simulink model "Mod3_4"  (Simulink 7.4)
settings: Solver=FixedStepDiscrete  SolverMode=SingleTasking  StartTime=0.0  StopTime=1  FixedStep=1/Fs  MaxStep=1e-6  RelTol=1e-3  AbsTol=1e-6
InitFcn:
  | Enable_Errors =0;
  | 
  | Alpha_ = Enable_Errors*[1e-3 1e-3 1e-3];        % integrator gain errors
  | Beta_  =  Enable_Errors*[ 1e-4  1e-4   1e-4];      % integrator pole error
  | 
  | if Enable_Errors==1
  |      C_gain = 1e5;   % comparitor gain
  | else
  |      C_gain=1e12;
  | end;
  | 
  | Fs_out = 100e3;   % output sample rate
  | OSR=64;               % input oversampling factor
  | Fs=OSR*Fs_out;   %  input sampling rate
undefined symbols (not defined in the file or in its folder): One, sided
libraries: simulink x4, dspbuff3 x3, dspsnks4 x2, dspmlti4 x2, dspspect3 x2, commsynccomp2 x1, dsparch4 x1, dspadpt3 x1, dspobslib x1, dspsigops x1, dspstat3 x1
settings Model: Creator=don  LastModifiedBy=Dick  ExtModeTrigMode=oneshot  ExtModeArmWhenConnect=off
settings DataIOCC: LimitDataPoints=off  SaveOutput=off  SaveTime=off  SignalLoggingName=sigsOut
settings OptimizationCC: BlockReduction=off  BooleanDataType=off  InitFltsAndDblsToZero=on
settings DebuggingCC: SaveWithParameterizedLinksMsg=none  SignalResolutionControl=TryResolveAllWithWarning  SolverPrmCheckMsg=none  MultiTaskDSMMsg=warning  MultiTaskCondExecSysMsg=none  IntegerOverflowMsg=none  StrictBusMsg=None
settings HardwareCC: TargetUnknown=on
settings RTWCC: IncludeERTFirstTime=on
settings GRTTargetCC: TargetFcnLib=ansi_tfl_tmw.mat

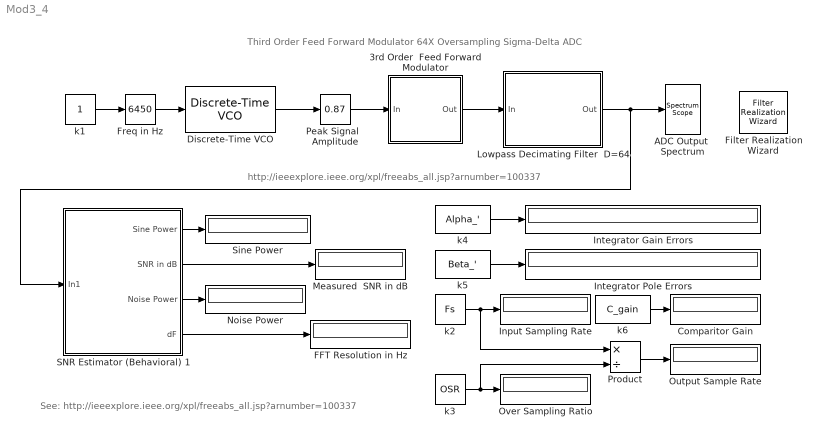
== system Mod3_4 ==
  note: Third Order Feed Forward Modulator
      | 64X Oversampling Sigma-Delta ADC
  note: http://ieeexplore.ieee.org/xpl/freeabs_all.jsp?arnumber=100337
  note: See: http://ieeexplore.ieee.org/xpl/freeabs_all.jsp?arnumber=100337
  3rd Order  Feed Forward Modulator : Subsystem
  ADC Output  Spectrum : dspsnks4/Spectrum Scope  DialogController=dspdialog.SpectrumScope  DialogControllerArgs=DataTag0  SystemSampleTime=-1  ScopeProperties=off  Domain=Frequency  HorizSpan=1  UseBuffer=on  BufferSize=1024  Overlap=0  inpFftLenInherit=off  FFTlength=128  numAvg=1  DisplayProperties=off  AxisGrid=on  Memory=off  FrameNumber=on  AxisLegend=off  AxisZoom=off  OpenScopeAtSimStart=on  OpenScopeImmediately=off  FigPos=[80 61 319 232]  AxisProperties=on  XUnits=Hertz  XRange=One-sided ([0...Fs/2])  XDisplay=0  InheritXIncr=on  XIncr=1.0  XLabel=Samples  XLimit=User-defined  YUnits=dBW  XMax=Fs/(2*OSR)  XMin=0  YLabel=Magnitude, dB  LineProperties=off  wintypeSpecScope=Hann  RsSpecScope=50  betaSpecScope=5  winsampSpecScope=Periodic  XAxisParamsVer=6.9
      settings: YMin=-200  YMax=0
  Comparitor Gain : Display
      settings: Decimation=1000
  Discrete-Time VCO : commsynccomp2/Discrete-Time VCO  SystemSampleTime=-1  Ac=1  Fc=0  Kc=1  Ph=0  ts=1/Fs
  FFT Resolution in Hz : Display
  Filter Realization Wizard : dsparch4/Filter Realization Wizard  SystemSampleTime=-1
  Freq in Hz : simulink/Math Operations/Slider Gain  SystemSampleTime=-1  low=0  gain=6450  high=20000
  Input Sampling Rate : Display
      settings: Decimation=1000
  Integrator Gain Errors : Display
      settings: Decimation=1000
  Integrator Pole Errors : Display
      settings: Decimation=1000
  Lowpass Decimating Filter  D=64 : Subsystem  Tag=BlockMethodSubSystem
  Measured  SNR in dB : Display
  Noise Power : Display
  Output Sample Rate : Display
      settings: Decimation=1000
  Over Sampling Ratio : Display
      settings: Decimation=1000
  Peak Signal   Amplitude : simulink/Math Operations/Slider Gain  SystemSampleTime=-1  low=0  gain=0.87  high=1
  Product : Product  Inputs=*/  OutDataType=fixdt(1, 16)  OutScaling=2^0  RndMeth=Zero
  SNR Estimator (Behavioral) 1 : Subsystem  mask{Frame=256, Pcnt_Nyquist=100, Navg=1, Ymax=-50, Ymin=-140, Hold_Off=260, ON_FFT_LINE=off}
      mask prompts: Frame "Input Frame Size"; Pcnt_Nyquist "Percentage of Fs/2 to use in noise power measurement"; Navg "Number of Averages"; Ymax "Noise Plot Ymax in dB"; Ymin "Noise Plot Ymin in dB"; Hold_Off "Calculation Hold Off in SAMPLES"; ON_FFT_LINE "Check this box if the signal is on an FFT Analysis Line."
      mask Display:
      | disp('SNR \n Measurement')
      | port_label('Input',1,'In')
      | port_label('Output',1,'Sine Power')
      | port_label('Output',2,'SNR in dB')
      | port_label('Output',3,'Noise Power')
      | port_label('Output',4,'FFT Line Freq')
  "Sine Power " : Display
  k1 : Constant  OutDataType=fixdt(1, 16)  OutScaling=2^0
  k2 : Constant  Value=Fs  OutDataType=fixdt(1, 16)  OutScaling=2^0
  k3 : Constant  Value=OSR  OutDataType=fixdt(1, 16)  OutScaling=2^0
  k4 : Constant  Value=Alpha_'  OutDataType=fixdt(1, 16)  OutScaling=2^0
  k5 : Constant  Value=Beta_'  OutDataType=fixdt(1, 16)  OutScaling=2^0
  k6 : Constant  Value=C_gain  OutDataType=fixdt(1, 16)  OutScaling=2^0
  wires:
  Discrete-Time VCO/1 -> Peak Signal   Amplitude/1
  Peak Signal   Amplitude/1 -> 3rd Order  Feed Forward Modulator/1(In)
  Freq in Hz/1 -> Discrete-Time VCO/1
  k1/1 -> Freq in Hz/1
  k3/1 -> Over Sampling Ratio/1, Product/2
  Product/1 -> Output Sample Rate/1
  Lowpass Decimating Filter  D=64/1(Out) -> ADC Output  Spectrum/1, SNR Estimator (Behavioral) 1/1(In1)
  SNR Estimator (Behavioral) 1/2(SNR in dB) -> Measured  SNR in dB/1
  SNR Estimator (Behavioral) 1/1(Sine Power) -> "Sine Power "/1
  SNR Estimator (Behavioral) 1/3(Noise Power) -> Noise Power/1
  SNR Estimator (Behavioral) 1/4(dF) -> FFT Resolution in Hz/1
  3rd Order  Feed Forward Modulator/1(Out) -> Lowpass Decimating Filter  D=64/1(In)
  k4/1 -> Integrator Gain Errors/1
  k5/1 -> Integrator Pole Errors/1
  k6/1 -> Comparitor Gain/1
  k2/1 -> Input Sampling Rate/1, Product/1

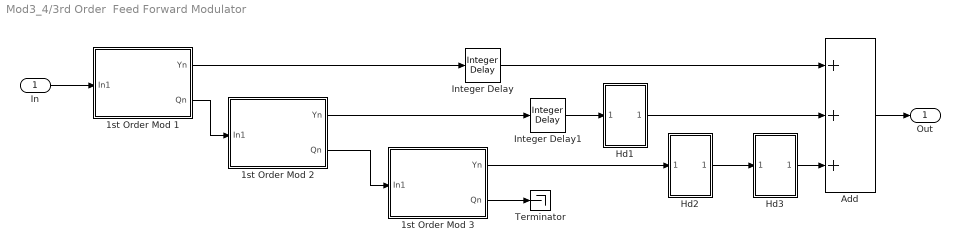
== system Mod3_4/3rd Order  Feed Forward Modulator ==
  In : Inport
  1st Order Mod 1 : Subsystem
  1st Order Mod 2 : Subsystem
  1st Order Mod 3 : Subsystem
  Add : Sum  Inputs=+++  OutDataType=fixdt(1, 16)  OutScaling=2^-10
  Hd1 : Subsystem
  Hd2 : Subsystem
  Hd3 : Subsystem
  Integer Delay : simulink/Discrete/Integer Delay  vinit=0.0  samptime=-1  NumDelays=2
  Integer Delay1 : simulink/Discrete/Integer Delay  vinit=0.0  samptime=-1  NumDelays=1
  Terminator : Terminator
  Out : Outport
  wires:
  1st Order Mod 1/2(Qn) -> 1st Order Mod 2/1(In1)
  1st Order Mod 2/2(Qn) -> 1st Order Mod 3/1(In1)
  1st Order Mod 1/1(Yn) -> Integer Delay/1
  Add/1 -> Out/1
  In/1 -> 1st Order Mod 1/1(In1)
  1st Order Mod 3/2(Qn) -> Terminator/1
  1st Order Mod 2/1(Yn) -> Integer Delay1/1
  Hd1/1(Out1) -> Add/2
  1st Order Mod 3/1(Yn) -> Hd2/1(In1)
  Hd2/1(Out1) -> Hd3/1(In1)
  Hd3/1(Out1) -> Add/3
  Integer Delay1/1 -> Hd1/1(In1)
  Integer Delay/1 -> Add/1

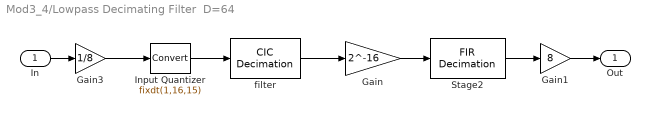
== system Mod3_4/Lowpass Decimating Filter  D=64 ==
  In : Inport
  Gain : Gain  Gain=2^-16  ParameterDataType=fixdt(1, 16)  ParameterScaling=2^0  OutDataTypeMode=double  OutDataType=fixdt(1, 16)  OutScaling=2^0  OutDataTypeStr=double
  Gain1 : Gain  Gain=8  ParameterDataType=fixdt(1, 16)  ParameterScaling=2^0  OutDataType=fixdt(1, 16)  OutScaling=2^0
  Gain3 : Gain  Gain=1/8  ParameterDataType=fixdt(1, 16)  ParameterScaling=2^0  OutDataType=fixdt(1, 16)  OutScaling=2^0
  Input Quantizer : DataTypeConversion  OutDataTypeMode=Specify via dialog  OutDataType=fixdt(1,16,15)  OutDataTypeStr=fixdt(1,16,15)  RndMeth=Round  SaturateOnIntegerOverflow=on
  Stage2 : dspmlti4/FIR Decimation  Tag=BlockMethodSubSystem  DialogController=dspdialog.FIRDecimation  DialogControllerArgs=DataTag1  h=[-1.03672832769806e-005 -2.30043872918871e-005 -3.81607660571471e-005 -4.73451966989753e-005 -4.15314840476983e-005 -1.53294381464531e-005 2.81247599902108e-005 7.548106001899e-005 0.000106956615554732 0.000105170685159055 6.53313671878897e-005 1.10615621617923e-006 -5.84899984530656e-005 -8.16995174647979e-005 -5.10738247202842e-005 2.39521887480776e-005 0.000107288371406307 0.000151796841211863 0.000124298000926512 2.72100582090589e-005 -9.64877715240933e-005 -0.000180990434728796 -0.00017184528528019 -5.94684973243738e-005 0.000107769129196385 0.000242056255586363 0.000260704715966674 0.00013493651668018 -8.5000049815582e-005 -0.000286841516056665 -0.000352051709584436 -0.000223619051276749 5.19058171754285e-005 0.000336492393063494 0.000467639101393255 0.000349059309073545 1.54942235654423e-005 -0.000369695852959625 -0.000591913524331285 -0.000502692833274323 -0.000114059879575764 0.000387970305599598 0.00072897644788482 0.000693620406886893 0.000257154373538894 -0.000377310868830626 -0.00086882045273623 -0.000918947560229279 -0.000448725221904726 0.000330696351510504 0.00100679796943566 0.00118065668729705 0.000698048038921545 -0.00023505915729049 -0.00113201638035961 -0.00147528588722154 -0.00101064908239849 7.91467137436565e-005 0.00123408252213311 0.00179975815120012 0.00139348389465366 0.000151247519594855 -0.00129860929748089 -0.00214716507990412 -0.00185109070890518 -0.000469898879291989 0.00131013209846719 0.00250931405838737 0.00238792045365338 0.000892372059188557 -0.00125000870520108 -0.00287487459601245 -0.00300688117971149 -0.00143501818412447 0.00109708430001496 0.00322994871994394 0.00371003867432686 0.00211584322619809 -0.000826876587517894 -0.00355768687459038 -0.00449894643382303 -0.00295548408089549 0.000410455632566669 0.00383775807505308 0.0053752440064593 0.00397885063139594 0.000187407314825939 -0.00404552680663259 -0.00634177196701517 -0.00521802991372615 -0.00101148845885873 0.00415062606771981 0.00740459885236922 0.00671755764137374 0.00212208484585908 -0.00411422714989155 -0.00857666811063853 -0.00854431755242137 -0.00360667248328686 0.00388301665917001 0.0098836881541225 0.0108056935767939 0.0056020971184406 -0.00337754872457966 -0.0113763732976555 -0.0136877273059045 -0.00834263488466605 0.00246546701482214 0.0131561884005966 0.0175416995656231 0.012273978356376 -0.000894329941755317 -0.0154384118477508 -0.0231117442236786 -0.0183702494962771 -0.00191023855567135 0.0187347462761574 0.0322678072014156 0.0292453606752335 0.00763813070524675 -0.0245476659764372 -0.0513189673918339 -0.0550085939173135 -0.0243158330095173 0.0395342433994632 0.121541322450517 0.197564379590681 0.24318839888947 0.24318839888947 0.197564379590681 0.121541322450517 0.0395342433994632 -0.0243158330095173 -0.0550085939173135 -0.0513189673918339 -0.0245476659764372 0.00763813070524675 0.0292453606752335 0.0322678072014156 0.0187347462761574 -0.00191023855567135 -0.0183702494962771 -0.0231117442236786 -0.0154384118477508 -0.000894329941755317 0.012273978356376 0.0175416995656231 0.0131561884005966 0.00246546701482214 -0.00834263488466605 -0.0136877273059045 -0.0113763732976555 -0.00337754872457966 0.0056020971184406 0.0108056935767939 0.0098836881541225 0.00388301665917001 -0.00360667248328686 -0.00854431755242137 -0.00857666811063853 -0.00411422714989155 0.00212208484585908 0.00671755764137374 0.00740459885236922 0.00415062606771981 -0.00101148845885873 -0.00521802991372615 -0.00634177196701517 -0.00404552680663259 0.000187407314825939 0.00397885063139594 0.0053752440064593 0.00383775807505308 0.000410455632566669 -0.00295548408089549 -0.00449894643382303 -0.00355768687459038 -0.000826876587517894 0.00211584322619809 0.00371003867432686 0.00322994871994394 0.00109708430001496 -0.00143501818412447 -0.00300688117971149 -0.00287487459601245 -0.00125000870520108 0.000892372059188557 0.00238792045365338 0.00250931405838737 0.00131013209846719 -0.000469898879291989 -0.00185109070890518 -0.00214716507990412 -0.00129860929748089 ...(+1336 chars)]  D=4  filtStruct=Direct form  framing=Maintain input frame size  outputBufInitCond=0  roundingMode=Floor  overflowMode=off  FilterSource=Specify via dialog  FilterObject=Hm_firdecim
  filter : dspmlti4/CIC Decimation  DialogController=dspdialog.CICDecimation  filtFrom=Dialog  filtobj=Hm_decim  ftype=Decimator  R=16  M=1  N=4  filterInternals=Full precision  BPS=[32 32 32 32 32 32 32 32]  FLPS=[15 15 15 15 15 15 15 15]  outputWordLength=32  outputFracLength=15  launchFVT=off  framing=Maintain input frame rate
  Out : Outport
  wires:
  In/1 -> Gain3/1
  filter/1 -> Gain/1
  Stage2/1 -> Gain1/1
  Gain/1 -> Stage2/1
  Gain1/1 -> Out/1
  Gain3/1 -> Input Quantizer/1
  Input Quantizer/1 -> filter/1

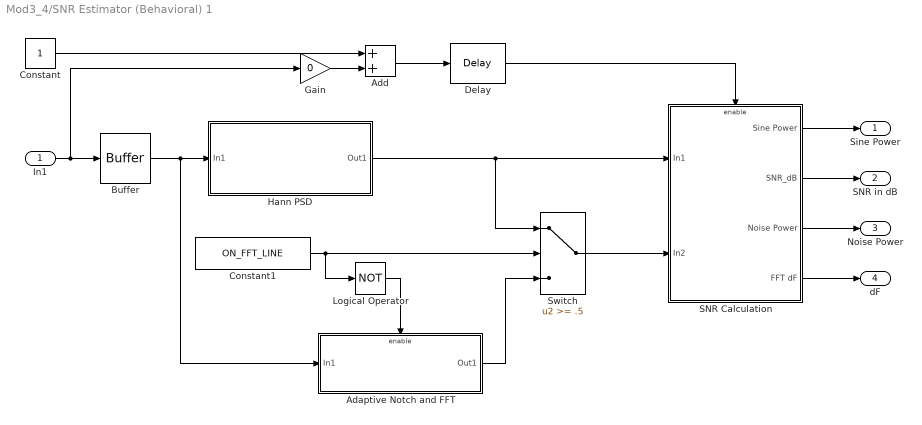
== system Mod3_4/SNR Estimator (Behavioral) 1 ==
  In1 : Inport
  Adaptive Notch and FFT : Subsystem  TreatAsAtomicUnit=on
  Add : Sum  OutDataType=fixdt(1, 16)  OutScaling=2^-10
  Buffer : dspbuff3/Buffer  N=Frame  V=0  ic=0
  Constant : Constant  OutDataType=fixdt(1, 16)  OutScaling=2^0
  Constant1 : Constant  Value=ON_FFT_LINE  OutDataTypeMode=boolean  OutDataType=fixdt(1, 16)  OutScaling=2^0  OutDataTypeStr=boolean
  Delay : dspsigops/Delay  dly_unit=Samples  delay=Hold_Off  ic_detail=off  dif_ic_for_ch=off  dif_ic_for_dly=off  ic=0  reset_popup=None
  Gain : Gain  Gain=0  ParameterDataType=fixdt(1, 16)  ParameterScaling=2^0  OutDataType=fixdt(1, 16)  OutScaling=2^0
  Hann PSD : Subsystem
  Logical Operator : Logic  Operator=NOT  AllPortsSameDT=off  OutDataTypeMode=boolean  LogicDataType=fixdt(0, 8)  OutDataTypeStr=boolean
  SNR Calculation : Subsystem
  Switch : Switch  Threshold=.5  OutDataType=fixdt(1, 16)  OutScaling=2^0
  Sine Power : Outport
  SNR in dB : Outport  Port=2
  Noise Power : Outport  Port=3
  dF : Outport  Port=4
  wires:
  In1/1 -> Buffer/1, Gain/1
  SNR Calculation/2(SNR_dB) -> SNR in dB/1
  Hann PSD/1(Out1) -> SNR Calculation/1(In1), Switch/1
  Buffer/1 -> Hann PSD/1(In1), Adaptive Notch and FFT/1(In1)
  SNR Calculation/1(Sine Power) -> Sine Power/1
  Switch/1 -> SNR Calculation/2(In2)
  SNR Calculation/3(Noise Power) -> Noise Power/1
  Delay/1 -> SNR Calculation/Enable
  Adaptive Notch and FFT/1(Out1) -> Switch/3
  Constant1/1 -> Switch/2, Logical Operator/1
  Logical Operator/1 -> Adaptive Notch and FFT/Enable
  SNR Calculation/4(FFT dF) -> dF/1
  Add/1 -> Delay/1
  Constant/1 -> Add/1
  Gain/1 -> Add/2

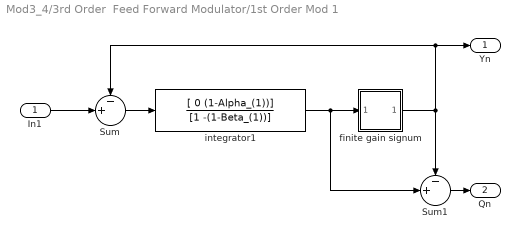
== system Mod3_4/3rd Order  Feed Forward Modulator/1st Order Mod 1 ==
  In1 : Inport
  Sum : Sum  Inputs=-+|  OutDataType=sfix(16)  OutScaling=2^0  SaturateOnIntegerOverflow=on  InputSameDT=on  OutDataTypeStr=Inherit: Same as first input
  Sum1 : Sum  Inputs=-+|  OutDataType=sfix(16)  OutScaling=2^0  SaturateOnIntegerOverflow=on  InputSameDT=on  OutDataTypeStr=Inherit: Same as first input
  "finite gain signum " : Subsystem  AncestorBlock=rab_favorites/non linear (real)  mask{alpha=C_gain}
      mask init:
      | x=-3:0.05:3;  y= tanh(alpha*x);
      mask Display: plot(x,y)
  integrator1 : DiscreteFilter  Numerator=[ 0 (1-Alpha_(1))]  Denominator=[1 -(1-Beta_(1))]
  Yn : Outport
  Qn : Outport  Port=2
  wires:
  Sum/1 -> integrator1/1
  integrator1/1 -> Sum1/2, "finite gain signum "/1(In1)
  Sum1/1 -> Qn/1
  "finite gain signum "/1(Out1) -> Sum1/1, Sum/1, Yn/1
  In1/1 -> Sum/2

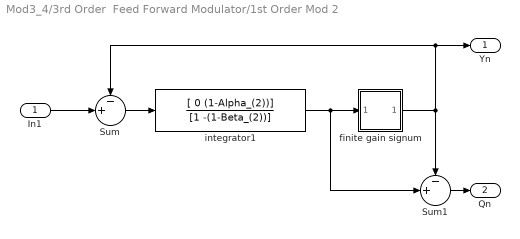
== system Mod3_4/3rd Order  Feed Forward Modulator/1st Order Mod 2 ==
  In1 : Inport
  Sum : Sum  Inputs=-+|  OutDataType=sfix(16)  OutScaling=2^0  SaturateOnIntegerOverflow=on  InputSameDT=on  OutDataTypeStr=Inherit: Same as first input
  Sum1 : Sum  Inputs=-+|  OutDataType=sfix(16)  OutScaling=2^0  SaturateOnIntegerOverflow=on  InputSameDT=on  OutDataTypeStr=Inherit: Same as first input
  "finite gain signum " : Subsystem  AncestorBlock=rab_favorites/non linear (real)  mask{alpha=C_gain}
      mask init:
      | x=-3:0.05:3;  y= tanh(alpha*x);
      mask Display: plot(x,y)
  integrator1 : DiscreteFilter  Numerator=[ 0 (1-Alpha_(2))]  Denominator=[1 -(1-Beta_(2))]
  Yn : Outport
  Qn : Outport  Port=2
  wires:
  In1/1 -> Sum/2
  "finite gain signum "/1(Out1) -> Yn/1, Sum/1, Sum1/1
  Sum1/1 -> Qn/1
  integrator1/1 -> "finite gain signum "/1(In1), Sum1/2
  Sum/1 -> integrator1/1

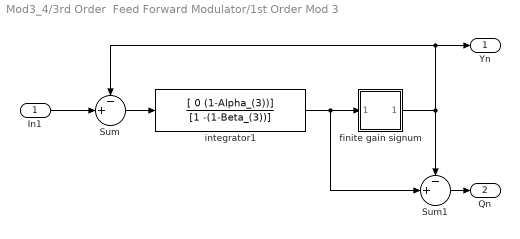
== system Mod3_4/3rd Order  Feed Forward Modulator/1st Order Mod 3 ==
  In1 : Inport
  Sum : Sum  Inputs=-+|  OutDataType=sfix(16)  OutScaling=2^0  SaturateOnIntegerOverflow=on  InputSameDT=on  OutDataTypeStr=Inherit: Same as first input
  Sum1 : Sum  Inputs=-+|  OutDataType=sfix(16)  OutScaling=2^0  SaturateOnIntegerOverflow=on  InputSameDT=on  OutDataTypeStr=Inherit: Same as first input
  "finite gain signum " : Subsystem  AncestorBlock=rab_favorites/non linear (real)  mask{alpha=C_gain}
      mask init:
      | x=-3:0.05:3;  y= tanh(alpha*x);
      mask Display: plot(x,y)
  integrator1 : DiscreteFilter  Numerator=[ 0 (1-Alpha_(3))]  Denominator=[1 -(1-Beta_(3))]
  Yn : Outport
  Qn : Outport  Port=2
  wires:
  Sum/1 -> integrator1/1
  integrator1/1 -> Sum1/2, "finite gain signum "/1(In1)
  Sum1/1 -> Qn/1
  "finite gain signum "/1(Out1) -> Sum1/1, Sum/1, Yn/1
  In1/1 -> Sum/2

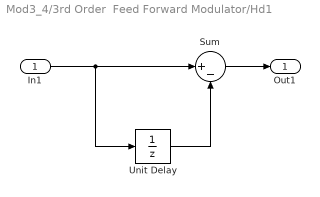
== system Mod3_4/3rd Order  Feed Forward Modulator/Hd1 ==
  In1 : Inport
  Sum : Sum  Inputs=|+-  OutDataType=sfix(16)  OutScaling=2^0  SaturateOnIntegerOverflow=on  InputSameDT=on  OutDataTypeStr=Inherit: Same as first input
  Unit Delay : UnitDelay  SampleTime=-1
  Out1 : Outport
  wires:
  In1/1 -> Sum/1, Unit Delay/1
  Sum/1 -> Out1/1
  Unit Delay/1 -> Sum/2

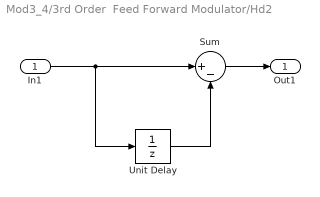
== system Mod3_4/3rd Order  Feed Forward Modulator/Hd2 ==
  In1 : Inport
  Sum : Sum  Inputs=|+-  OutDataType=sfix(16)  OutScaling=2^0  SaturateOnIntegerOverflow=on  InputSameDT=on  OutDataTypeStr=Inherit: Same as first input
  Unit Delay : UnitDelay  SampleTime=-1
  Out1 : Outport
  wires:
  Unit Delay/1 -> Sum/2
  Sum/1 -> Out1/1
  In1/1 -> Unit Delay/1, Sum/1

== system Mod3_4/3rd Order  Feed Forward Modulator/Hd3 ==
  In1 : Inport
  Sum : Sum  Inputs=|+-  OutDataType=sfix(16)  OutScaling=2^0  SaturateOnIntegerOverflow=on  InputSameDT=on  OutDataTypeStr=Inherit: Same as first input
  Unit Delay : UnitDelay  SampleTime=-1
  Out1 : Outport
  wires:
  In1/1 -> Sum/1, Unit Delay/1
  Sum/1 -> Out1/1
  Unit Delay/1 -> Sum/2

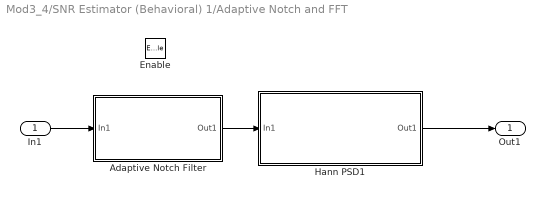
== system Mod3_4/SNR Estimator (Behavioral) 1/Adaptive Notch and FFT ==
  In1 : Inport  OutDataType=fixdt(1, 16)  OutScaling=2^0
  Enable : EnablePort
  Adaptive Notch Filter : Subsystem
  Hann PSD1 : Subsystem
  Out1 : Outport  OutDataType=fixdt(1, 16)  OutScaling=2^0
  wires:
  Adaptive Notch Filter/1(Out1) -> Hann PSD1/1(In1)
  Hann PSD1/1(Out1) -> Out1/1
  In1/1 -> Adaptive Notch Filter/1(In1)

== system Mod3_4/SNR Estimator (Behavioral) 1/Hann PSD ==
  note: Real Data produces a perfectly
      | symmetrical spectrum.
      | Use 1/2 of it.
  In1 : Inport
  Periodogram using  Hann Window : dspspect3/Periodogram  SystemSampleTime=-1  measurement=Mean-square spectrum  wintype=Hann  Rs=RsSpecScope  beta=betaSpecScope  winsamp=Periodic  inheritFFT=on  fftsize=FFTlength  navg=Navg  inheritTs=on  Ts=1
  Selector : Selector  InputPortWidth=Frame  IndexOptions=Index vector (dialog)  Indices=[1: Frame/2]  OutputSizes=1
  Out1 : Outport
  wires:
  Selector/1 -> Out1/1
  Periodogram using  Hann Window/1 -> Selector/1
  In1/1 -> Periodogram using  Hann Window/1

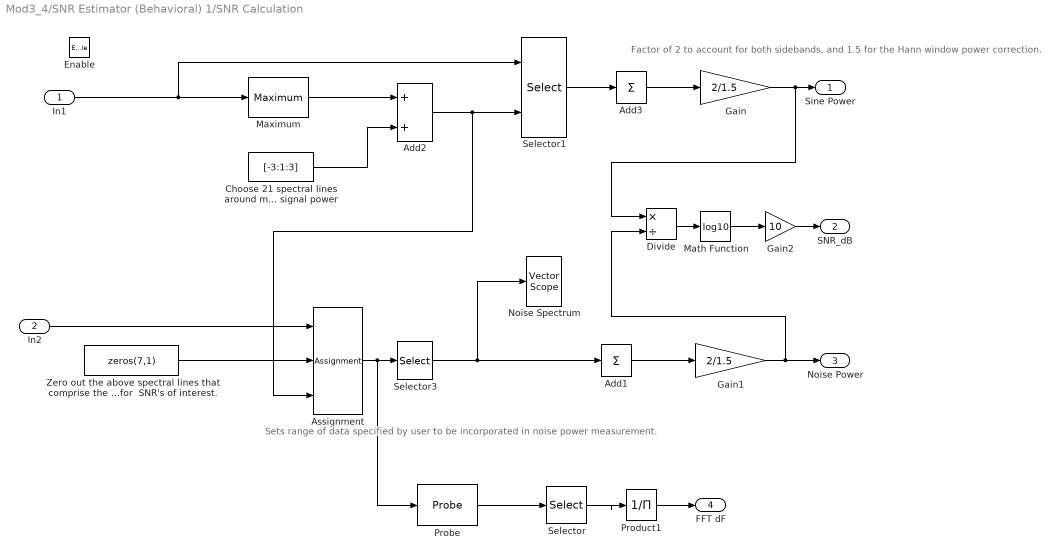
== system Mod3_4/SNR Estimator (Behavioral) 1/SNR Calculation ==
  note: Factor of 2 to account for both sidebands,
      | and 1.5 for the Hann window
      | power correction.
  note: Sets range of data
      | specified by user to be
      |  incorporated in
      | noise power measurement.
  In1 : Inport
  In2 : Inport  Port=2
  Enable : EnablePort
  Add1 : Sum  Inputs=+  OutDataType=fixdt(1, 16)  OutScaling=2^-10
  Add2 : Sum  OutDataType=fixdt(1, 16)  OutScaling=2^-10
  Add3 : Sum  Inputs=+  OutDataType=fixdt(1, 16)  OutScaling=2^-10
  Assignment : Assignment  IndexOptions=Index vector (port)  Indices=1  OutputSizes=1
  Choose 21 spectral lines around max to  estimate signal power : Constant  Value=[-3:1:3]  OutDataType=fixdt(1, 16)  OutScaling=2^0
  Divide : Product  Inputs=*/  OutDataType=fixdt(1, 16)  OutScaling=2^-10
  Gain : Gain  Gain=2/1.5  ParameterDataType=fixdt(1, 16)  ParameterScaling=2^0  OutDataType=fixdt(1, 16)  OutScaling=2^0
  Gain1 : Gain  Gain=2/1.5  ParameterDataType=fixdt(1, 16)  ParameterScaling=2^0  OutDataType=fixdt(1, 16)  OutScaling=2^0
  Gain2 : Gain  Gain=10  ParameterDataType=fixdt(1, 16)  ParameterScaling=2^0  OutDataType=fixdt(1, 16)  OutScaling=2^0
  Math Function : Math  Operator=log10  OutDataType=fixdt(1, 16)  OutScaling=2^0  SaturateOnIntegerOverflow=on
  Maximum : dspstat3/Maximum  DialogController=dspDDGCreate  DialogControllerArgs=DataTag2  fcn=Index  reset=None  indexBase=One  operateOver=Each column  Dimension=1  colComp=on  operation=maximum  roiEnable=off  roiType=Rectangles  roiPortion=Entire ROI  roiOutput=Individual statistics for each ROI  roiFlag=off  accumDataTypeStr=Inherit: Same as product output  accumLastDataTypeStr=Inherit: Same as product output  roundingMode=Floor  overflowMode=off
  Noise Spectrum : dspsnks4/Vector Scope  DialogController=dspdialog.VectorScope  DialogControllerArgs=DataTag3  ScopeProperties=on  Domain=Frequency  HorizSpan=1  DisplayProperties=off  AxisGrid=on  Memory=off  FrameNumber=on  AxisLegend=off  AxisZoom=off  OpenScopeAtSimStart=on  OpenScopeImmediately=off  FigPos=[755 36 259 173]  AxisProperties=off  XUnits=Hertz  XRange=[0...Fs]  InheritXIncr=on  XIncr=1  XLabel=Time  XLimit=Auto  XMin=0  XMax=50000  XStart=0  YUnits=dB  YLabel=dBW  LineProperties=off  XAxisParamsVer=6.9
      settings: YMin=Ymin  YMax=Ymax
  Probe : Probe  ProbeWidth=off  ProbeComplexSignal=off
  Product1 : Product  Inputs=/  OutDataType=fixdt(1, 16)  OutScaling=2^0  RndMeth=Zero
  Selector : Selector  InputPortWidth=2  IndexOptions=Index vector (dialog)  Indices=1  OutputSizes=1
  Selector1 : Selector  InputPortWidth=Frame/2  IndexOptions=Index vector (port)  Indices=[1: Frame/2]  OutputSizes=1
  Selector3 : Selector  InputPortWidth=Frame/2  IndexOptions=Index vector (dialog)  Indices=[1: round(Pcnt_Nyquist*Frame/200)]  OutputSizes=1
  "Zero out the above spectral lines that comprise the signal. Zeroing should not induce any significant error for  SNR's of interest. " : Constant  Value=zeros(7,1)  OutDataType=fixdt(1, 16)  OutScaling=2^0
  Sine Power : Outport
  SNR_dB : Outport  Port=2
  Noise Power : Outport  Port=3
  FFT dF : Outport  Port=4
  wires:
  "Zero out the above spectral lines that comprise the signal. Zeroing should not induce any significant error for  SNR's of interest. "/1 -> Assignment/2
  Add1/1 -> Gain1/1
  Add3/1 -> Gain/1
  Divide/1 -> Math Function/1
  Math Function/1 -> Gain2/1
  Maximum/1 -> Add2/1
  Choose 21 spectral lines around max to  estimate signal power/1 -> Add2/2
  Add2/1 -> Selector1/2, Assignment/3
  Selector1/1 -> Add3/1
  Selector3/1 -> Add1/1, Noise Spectrum/1
  In2/1 -> Assignment/1
  In1/1 -> Maximum/1, Selector1/1
  Gain2/1 -> SNR_dB/1
  Gain/1 -> Divide/1, Sine Power/1
  Gain1/1 -> Divide/2, Noise Power/1
  Assignment/1 -> Selector3/1, Probe/1
  Probe/1 -> Selector/1
  Selector/1 -> Product1/1
  Product1/1 -> FFT dF/1

== system Mod3_4/3rd Order  Feed Forward Modulator/1st Order Mod 1/finite gain signum  ==
  In1 : Inport  OutDataType=sfix(16)  OutScaling=2^0
  Gain1 : Gain  Gain=alpha  ParameterDataType=sfix(16)  ParameterScaling=2^0  OutDataType=sfix(16)  OutScaling=2^0  SaturateOnIntegerOverflow=on  OutDataTypeStr=Inherit: Same as input  ParamDataTypeStr=Inherit: Same as input
  Hyperbolic Tangent : Trigonometry  Operator=tanh
  Out1 : Outport  OutDataType=sfix(16)  OutScaling=2^0
  wires:
  Hyperbolic Tangent/1 -> Out1/1
  Gain1/1 -> Hyperbolic Tangent/1
  In1/1 -> Gain1/1

== system Mod3_4/3rd Order  Feed Forward Modulator/1st Order Mod 2/finite gain signum  ==
  In1 : Inport  OutDataType=sfix(16)  OutScaling=2^0
  Gain1 : Gain  Gain=alpha  ParameterDataType=sfix(16)  ParameterScaling=2^0  OutDataType=sfix(16)  OutScaling=2^0  SaturateOnIntegerOverflow=on  OutDataTypeStr=Inherit: Same as input  ParamDataTypeStr=Inherit: Same as input
  Hyperbolic Tangent : Trigonometry  Operator=tanh
  Out1 : Outport  OutDataType=sfix(16)  OutScaling=2^0
  wires:
  In1/1 -> Gain1/1
  Gain1/1 -> Hyperbolic Tangent/1
  Hyperbolic Tangent/1 -> Out1/1

== system Mod3_4/3rd Order  Feed Forward Modulator/1st Order Mod 3/finite gain signum  ==
  In1 : Inport  OutDataType=sfix(16)  OutScaling=2^0
  Gain1 : Gain  Gain=alpha  ParameterDataType=sfix(16)  ParameterScaling=2^0  OutDataType=sfix(16)  OutScaling=2^0  SaturateOnIntegerOverflow=on  OutDataTypeStr=Inherit: Same as input  ParamDataTypeStr=Inherit: Same as input
  Hyperbolic Tangent : Trigonometry  Operator=tanh
  Out1 : Outport  OutDataType=sfix(16)  OutScaling=2^0
  wires:
  Hyperbolic Tangent/1 -> Out1/1
  Gain1/1 -> Hyperbolic Tangent/1
  In1/1 -> Gain1/1

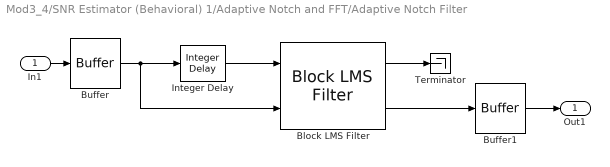
== system Mod3_4/SNR Estimator (Behavioral) 1/Adaptive Notch and FFT/Adaptive Notch Filter ==
  In1 : Inport
  Block LMS Filter : dspadpt3/Block LMS Filter  algo=Block LMS  L=20  N=64  stepflag=Dialog  mu=0.005  leakage=.99999  addnparflag=on  ic=0  Adapt=off  resetflag=None  weights=off
  Buffer : dspbuff3/Buffer  N=64  V=0  ic=0
  Buffer1 : dspbuff3/Buffer  N=Frame  V=0  ic=0
  Integer Delay : dspobslib/Integer Delay  delay=10  ic=0  reset_popup=None
  Terminator : Terminator
  Out1 : Outport
  wires:
  Block LMS Filter/1 -> Terminator/1
  Block LMS Filter/2 -> Buffer1/1
  Buffer1/1 -> Out1/1
  In1/1 -> Buffer/1
  Buffer/1 -> Block LMS Filter/2, Integer Delay/1
  Integer Delay/1 -> Block LMS Filter/1

== system Mod3_4/SNR Estimator (Behavioral) 1/Adaptive Notch and FFT/Hann PSD1 ==
  note: Real Data produces a perfectly
      | symmetrical spectrum.
      | Use 1/2 of it.
  In1 : Inport
  Periodogram using  Hann Window : dspspect3/Periodogram  SystemSampleTime=-1  measurement=Mean-square spectrum  wintype=Hann  Rs=RsSpecScope  beta=betaSpecScope  winsamp=Periodic  inheritFFT=on  fftsize=FFTlength  navg=Navg  inheritTs=on  Ts=1
  Selector : Selector  InputPortWidth=Frame  IndexOptions=Index vector (dialog)  Indices=[1: Frame/2]  OutputSizes=1
  Out1 : Outport
  wires:
  In1/1 -> Periodogram using  Hann Window/1
  Periodogram using  Hann Window/1 -> Selector/1
  Selector/1 -> Out1/1
